simulink model "tp1_2"  (R2023b)
settings: Solver=VariableStepAuto  StartTime=0.0  StopTime=30  RelTol=1e-3
settings Model: Creator=rusha  LastModifiedBy=rusha

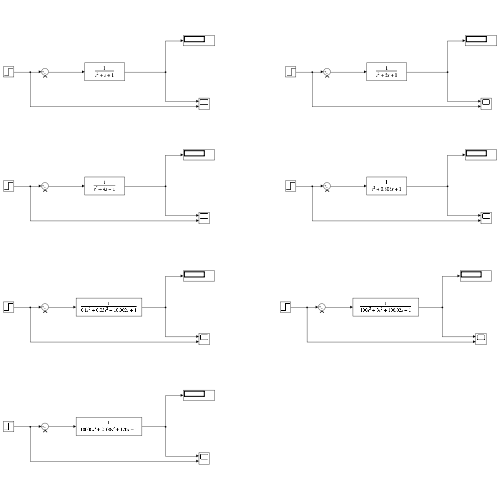
[thumbnail: Simulink's stored preview of the top-level diagram]
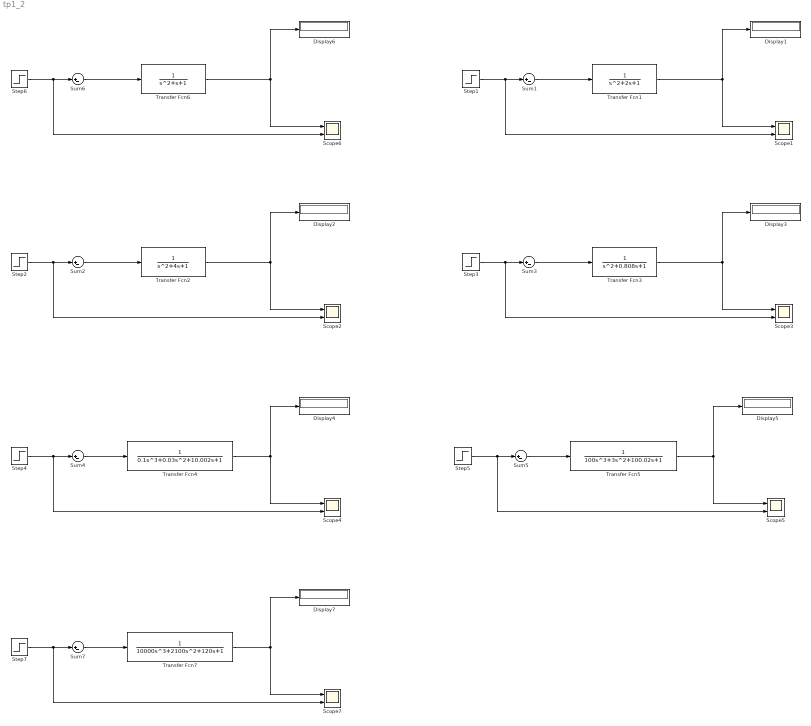
== system tp1_2 ==
  Display{1..7} (7 alike) : Display
  Scope{1..7} (7 alike) : Scope  NumInputPorts=2
  Step{1..7} (7 alike) : Step  SampleTime=0
  Sum{1..7} (7 alike) : Sum  Inputs=|+-
  Transfer Fcn1 : TransferFcn
  Transfer Fcn2 : TransferFcn  Denominator=[1 4 1]
  Transfer Fcn3 : TransferFcn  Denominator=[1 0.808 1]
  Transfer Fcn4 : TransferFcn  Denominator=[0.1 0.03 10.002 1]
  Transfer Fcn5 : TransferFcn  Denominator=[100 3 100.02 1]
  Transfer Fcn6 : TransferFcn  Denominator=[1 1 1]
  Transfer Fcn7 : TransferFcn  Denominator=[10000 2100 120 1]
  wires:
  Sum6/1 -> Transfer Fcn6/1
  Step6/1 -> Scope6/2, Sum6/1
  Transfer Fcn6/1 -> Display6/1, Scope6/1
  Step1/1 -> Scope1/2, Sum1/1
  Transfer Fcn1/1 -> Display1/1, Scope1/1
  Sum1/1 -> Transfer Fcn1/1
  Step2/1 -> Scope2/2, Sum2/1
  Transfer Fcn2/1 -> Display2/1, Scope2/1
  Sum2/1 -> Transfer Fcn2/1
  Step3/1 -> Scope3/2, Sum3/1
  Transfer Fcn3/1 -> Display3/1, Scope3/1
  Sum3/1 -> Transfer Fcn3/1
  Step4/1 -> Scope4/2, Sum4/1
  Transfer Fcn4/1 -> Display4/1, Scope4/1
  Sum4/1 -> Transfer Fcn4/1
  Sum5/1 -> Transfer Fcn5/1
  Transfer Fcn5/1 -> Display5/1, Scope5/1
  Step5/1 -> Scope5/2, Sum5/1
  Sum7/1 -> Transfer Fcn7/1
  Transfer Fcn7/1 -> Display7/1, Scope7/1
  Step7/1 -> Scope7/2, Sum7/1
